simulink subsystem "quatConventionConverter"  (R2025b)
settings: Solver=VariableStepAuto  StartTime=0.0  StopTime=10.0  RelTol=1e-3
model mask{conversion=q0 to q4}
settings Model: Creator=antoniohernandez-rodiciomateos  LastModifiedBy=antoniohernandez-rodiciomateos

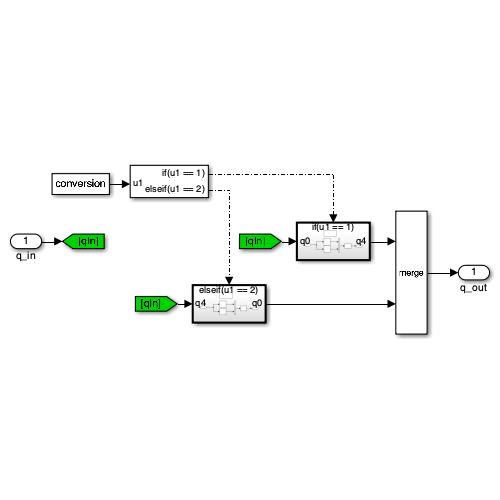
[thumbnail: Simulink's stored preview of the top-level diagram]
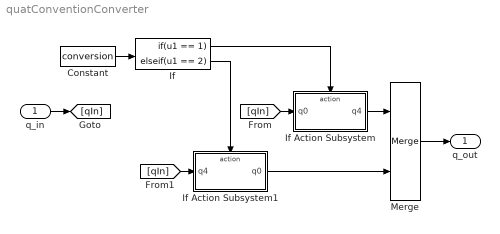
== system quatConventionConverter ==
  q_in : Inport  PortDimensions=[4 1]
  Constant : Constant  Value=conversion
  If : If  IfExpression=u1 == 1  ElseIfExpressions=u1 == 2  ShowElse=off
  If Action Subsystem : Subsystem  TreatAsAtomicUnit=on
  If Action Subsystem1 : Subsystem  TreatAsAtomicUnit=on
  Merge : Merge
  q_out : Outport  PortDimensions=[4 1]
  wires:
  Constant/1 -> If/1
  If/1 -> If Action Subsystem/Action
  q_in/1 -> [qIn]
  If/2 -> If Action Subsystem1/Action
  If Action Subsystem/1(q4) -> Merge/1
  If Action Subsystem1/1(q0) -> Merge/2
  [qIn] -> If Action Subsystem/1(q0)
  [qIn] -> If Action Subsystem1/1(q4)
  Merge/1 -> q_out/1

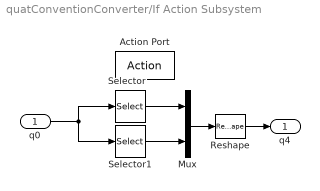
== system quatConventionConverter/If Action Subsystem ==
  q0 : Inport  PortDimensions=[4 1]
  Action Port : ActionPort  ActionPortLabel=if(u1 == 1)
  Mux : Mux  Inputs=2
  Reshape : Reshape  OutputDimensionality=Column vector (2-D)
  Selector : Selector  InputPortWidth=4  IndexOptions=Index vector (dialog)  Indices=[2 3 4]  OutputSizes=1
  Selector1 : Selector  InputPortWidth=4  IndexOptions=Index vector (dialog)  Indices=[1]  OutputSizes=1
  q4 : Outport  PortDimensions=[4 1]
  wires:
  Selector/1 -> Mux/1
  Selector1/1 -> Mux/2
  q0/1 -> Selector1/1, Selector/1
  Mux/1 -> Reshape/1
  Reshape/1 -> q4/1

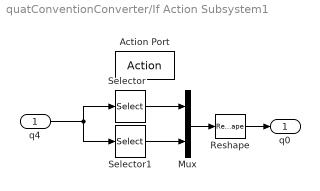
== system quatConventionConverter/If Action Subsystem1 ==
  q4 : Inport  PortDimensions=[4 1]
  Action Port : ActionPort  ActionPortLabel=elseif(u1 == 2)
  Mux : Mux  Inputs=2
  Reshape : Reshape  OutputDimensionality=Column vector (2-D)
  Selector : Selector  InputPortWidth=4  IndexOptions=Index vector (dialog)  Indices=[4]  OutputSizes=1
  Selector1 : Selector  InputPortWidth=4  IndexOptions=Index vector (dialog)  Indices=[1 2 3]  OutputSizes=1
  q0 : Outport  PortDimensions=[4 1]
  wires:
  Selector/1 -> Mux/1
  Selector1/1 -> Mux/2
  Mux/1 -> Reshape/1
  Reshape/1 -> q0/1
  q4/1 -> Selector1/1, Selector/1
